simulink library "threeThrSP_cl"  (R2018b)
settings: Solver=VariableStepAuto  StartTime=0.0  StopTime=10.0  RelTol=1e-3
undefined symbols (not defined in the file): rollAmp, startRoll
settings Model: Creator=asiddiq2  LastModifiedBy=asiddiq2

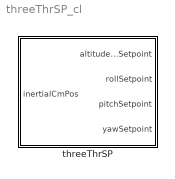
== system threeThrSP_cl ==
  threeThrSP : Subsystem

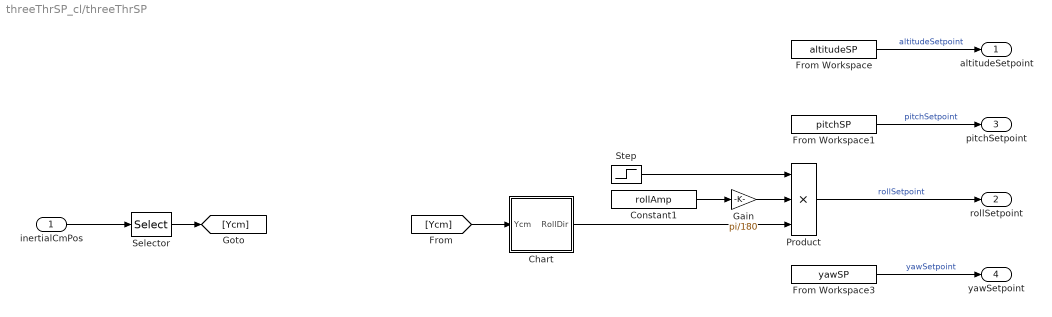
== system threeThrSP_cl/threeThrSP ==
  inertialCmPos : Inport
  Chart : Stateflow chart  TreatAsAtomicUnit=on
  Constant1 : Constant  Value=rollAmp
  From Workspace : FromWorkspace  VariableName=altitudeSP  SampleTime=0
  From Workspace1 : FromWorkspace  VariableName=pitchSP  SampleTime=0
  From Workspace3 : FromWorkspace  VariableName=yawSP  SampleTime=0
  Gain : Gain  Gain=pi/180
  Product : Product  Inputs=3
  Selector : Selector  InputPortWidth=3  IndexOptions=Index vector (dialog)  Indices=2  OutputSizes=1
  Step : Step  Time=startRoll  SampleTime=0
  altitudeSetpoint : Outport
  rollSetpoint : Outport  Port=2
  pitchSetpoint : Outport  Port=3
  yawSetpoint : Outport  Port=4
  wires:
  inertialCmPos/1 -> Selector/1
  Selector/1 -> [Ycm]
  Gain/1 -> Product/2
  Constant1/1 -> Gain/1
  Chart/1(RollDir) -> Product/3
  [Ycm] -> Chart/1(Ycm)
  Product/1 -> rollSetpoint/1  "rollSetpoint"
  From Workspace1/1 -> pitchSetpoint/1  "pitchSetpoint"
  From Workspace3/1 -> yawSetpoint/1  "yawSetpoint"
  From Workspace/1 -> altitudeSetpoint/1  "altitudeSetpoint"
  Step/1 -> Product/1

== stateflow chart threeThrSP_cl/threeThrSP/Chart ==
  state Positive_roll
    entry:
    RollDir = 1;
  state Negative_roll
    entry:
    RollDir = -1;
  (default) -> Positive_roll
  Negative_roll -> Positive_roll : [Ycm>Yswitch]
  Positive_roll -> Negative_roll : [Ycm<-Yswitch]
  data: Ycm input; Yswitch parameter; RollDir output
